simulink model "sistema_realimentado_sin_controlador"  (Simulink 7.7)
settings: Solver=ode3  StartTime=0.0  StopTime=20.0  FixedStep=0.01  RelTol=1e-3
libraries: simulink x1
settings Model: Creator=juen  LastModifiedBy=juen
settings DataIOCC: LimitDataPoints=off

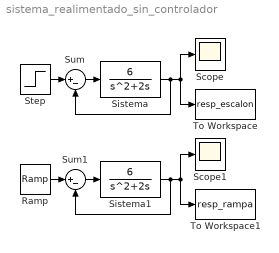
== system sistema_realimentado_sin_controlador ==
  Ramp : simulink/Sources/Ramp  SystemSampleTime=-1  slope=1  start=0  X0=0
  Scope : Scope
  Scope1 : Scope
  Sistema : TransferFcn  Numerator=[6]  Denominator=[1 2 0]
  Sistema1 : TransferFcn  Numerator=[6]  Denominator=[1 2 0]
  Step : Step  SampleTime=0
  Sum : Sum  Inputs=|+-
  Sum1 : Sum  Inputs=|+-
  To Workspace : ToWorkspace  VariableName=resp_escalon  SampleTime=-1  SaveFormat=Structure With Time
  To Workspace1 : ToWorkspace  VariableName=resp_rampa  SampleTime=-1  SaveFormat=Structure With Time
  wires:
  Step/1 -> Sum/1
  Sistema/1 -> Scope/1, To Workspace/1, Sum/2
  Sum/1 -> Sistema/1
  Ramp/1 -> Sum1/1
  Sistema1/1 -> Scope1/1, To Workspace1/1, Sum1/2
  Sum1/1 -> Sistema1/1
